simulink model "e01"  (R2023b)
settings: Solver=VariableStepAuto  StartTime=0.0  StopTime=10.0  RelTol=1e-3
values from neighbouring files (symbols this model uses):
  A = [ ... (first row only)    [e00.m]
  B = [ ... (first row only)    [e00.m]
  C = [ ... (first row only)    [e00.m]
  D = [ ... (first row only)    [e00.m]
  Ts = 0.5    [e00.m]
settings Model: Creator=jitbi  LastModifiedBy=Anirvan Krishna

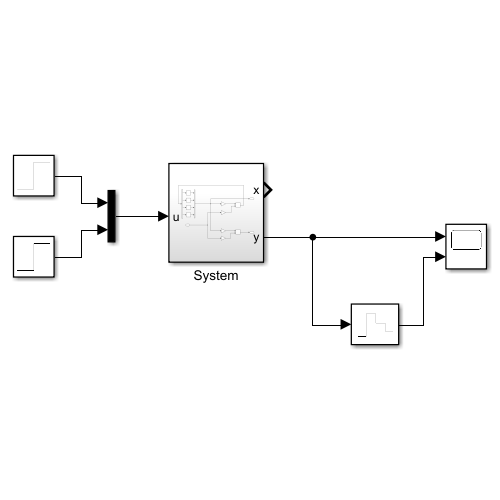
[thumbnail: Simulink's stored preview of the top-level diagram]
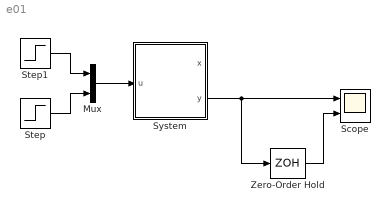
== system e01 ==
  Mux : Mux  Inputs=2
  Scope : Scope  NumInputPorts=2
  Step : Step  Time=0  SampleTime=1e-4
  Step1 : Step  Time=0  SampleTime=1e-4
  System : Subsystem
  Zero-Order Hold : ZeroOrderHold  SampleTime=Ts
  wires:
  Mux/1 -> System/1(u)
  System/2(y) -> Scope/1, Zero-Order Hold/1
  Zero-Order Hold/1 -> Scope/2
  Step1/1 -> Mux/1
  Step/1 -> Mux/2

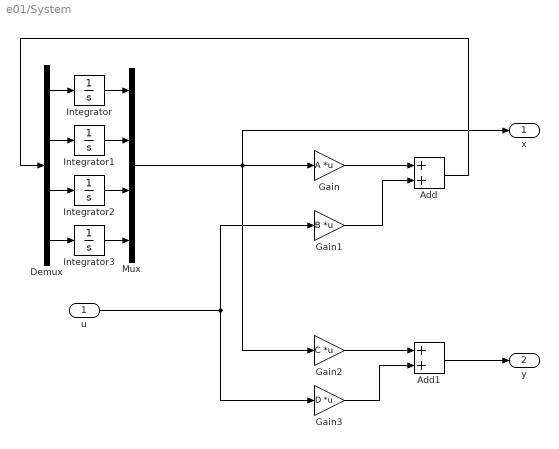
== system e01/System ==
  u : Inport
  Add : Sum
  Add1 : Sum
  Demux : Demux
  Gain : Gain  Gain=A  Multiplication=Matrix(K*u)
  Gain1 : Gain  Gain=B  Multiplication=Matrix(K*u)
  Gain2 : Gain  Gain=C  Multiplication=Matrix(K*u)
  Gain3 : Gain  Gain=D  Multiplication=Matrix(K*u)
  Integrator{,1..3} (4 alike) : Integrator
  Mux : Mux
  x : Outport
  y : Outport  Port=2
  wires:
  Demux/1 -> Integrator/1
  Gain3/1 -> Add1/2
  Integrator/1 -> Mux/1
  u/1 -> Gain3/1, Gain1/1
  Add/1 -> Demux/1
  Demux/3 -> Integrator2/1
  Integrator2/1 -> Mux/3
  Mux/1 -> x/1, Gain/1, Gain2/1
  Demux/4 -> Integrator3/1
  Demux/2 -> Integrator1/1
  Integrator3/1 -> Mux/4
  Integrator1/1 -> Mux/2
  Gain2/1 -> Add1/1
  Gain/1 -> Add/1
  Gain1/1 -> Add/2
  Add1/1 -> y/1
